simulink model "example_WeatherDatafile_inSubsystem"  (R2018b)
settings: Solver=ode45  StartTime=0.0  StopTime=24*3600  RelTol=1e-3  EnableMultiTasking=on
undefined symbols (not defined in the file): path_carnot
libraries: carnot x2
settings Model: Creator=drhf  LastModifiedBy=drhf
settings DataIOCC: LimitDataPoints=on  SaveFormat=Array
settings OptimizationCC: ExpressionDepthLimit=2147483647  LifeSpan=inf
settings DebuggingCC: UnderspecifiedInitializationDetection=Classic  MergeDetectMultiDrivingBlocksExec=none  StateNameClashWarn=warning  SFUnexpectedBacktrackingDiag=warning  SFNoUnconditionalDefaultTransitionDiag=warning  SFExecutionAtInitializationDiag=none
settings HardwareCC: ProdBitPerPointer=32  ProdBitPerSizeT=32  ProdBitPerPtrDiffT=32  ProdLargestAtomicFloat=None  ProdIntDivRoundTo=Undefined  ProdEndianess=Unspecified  ProdWordSize=32  ProdHWDeviceType=32-bit Generic
settings ModelReferenceCC: PropagateSignalLabelsOutOfModel=off
settings SFSimCC: SimUseLocalCustomCode=off
settings RTWCC: RTWUseLocalCustomCode=off
settings CodeAppCC: StateflowObjectComments=on
settings GRTTargetCC: TargetLangStandard=C89/C90 (ANSI)  GeneratePreprocessorConditionals=Disable all  CombineOutputUpdateFcns=off  GRTInterface=on
settings ConfigComp: CovMetricSettings=dw  CovHtmlReporting=on  CovSaveCumulativeToWorkspaceVar=on  CovSaveSingleToWorkspaceVar=on  CovExternalEMLEnable=off

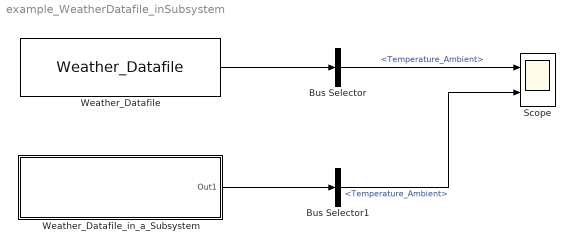
== system example_WeatherDatafile_inSubsystem ==
  Bus Selector : BusSelector  OutputSignals=Temperature_Ambient
  Bus Selector1 : BusSelector  OutputSignals=Temperature_Ambient
  Scope : Scope  NumInputPorts=2
  Weather_Datafile : carnot/Weather/Weather_Datafile  PathName=path_carnot('data')  FileName='DE_TRY2010_06_averageYear.mat'  UserParam=off  VariableName=DE_TRY2010_06_averageYear  SampleTime=3600
  Weather_Datafile_in_a_Subsystem : Subsystem  mask{PathName=path_carnot('data'), FileName='DE_TRY2010_06_averageYear.mat'}
      mask prompts: PathName "Selected path"; FileName "File"
      mask TypeOptions PathName: Weather_Datafile/PathName
      mask TypeOptions FileName: Weather_Datafile/FileName
  wires:
  Weather_Datafile/1 -> Bus Selector/1
  Bus Selector/1 -> Scope/1  "<Temperature_Ambient>"
  Bus Selector1/1 -> Scope/2  "<Temperature_Ambient>"
  Weather_Datafile_in_a_Subsystem/1(Out1) -> Bus Selector1/1

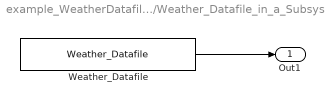
== system example_WeatherDatafile_inSubsystem/Weather_Datafile_in_a_Subsystem ==
  Weather_Datafile : carnot/Weather/Weather_Datafile  PathName=PathName  FileName=FileName  UserParam=off  VariableName=DE_TRY2010_06_averageYear  SampleTime=3600
  Out1 : Outport
  wires:
  Weather_Datafile/1 -> Out1/1
